simulink model "l1ipswing"  (Simulink 5.0)
settings: Solver=ode1  SolverMode=SingleTasking  StartTime=0.0  StopTime=inf  FixedStep=0.005  RelTol=1e-3
settings Model: LastModifiedBy=Administrator  ExtModeMexFile=rtwinext  ExtModeTrigDuration=100000  SimulationMode=external  LimitDataPoints=off  MaxDataPoints=20000  RTWSystemTargetFile=rtwin.tlc  RTWTemplateMakefile=rtwintmf  RTWOptions="-aCCOptimize=1 -aEnforceIntegerDowncast=1 -aExtMode=1 -aFoldNonRolledExpr=1 -aForceParamTrailComments=0 -aGenerateComments=1 -aGenerateReport=0 -aIncDataTypeInIds=0 -aIncHierarchyInIds=0 -aInlineInvariantSignals=0 -aInlineParameters=0 -aInlinedPrmAccess=\"Literals\" -aLocalBlockOutputs=1 -aMaxRTWIdLen=31 -aPrefixModelToSubsysFcnNames=1 -aRTWVerbose=1 -aRebuildAll=0 -aRollThreshold=5 -aShowEliminatedStatements=0"

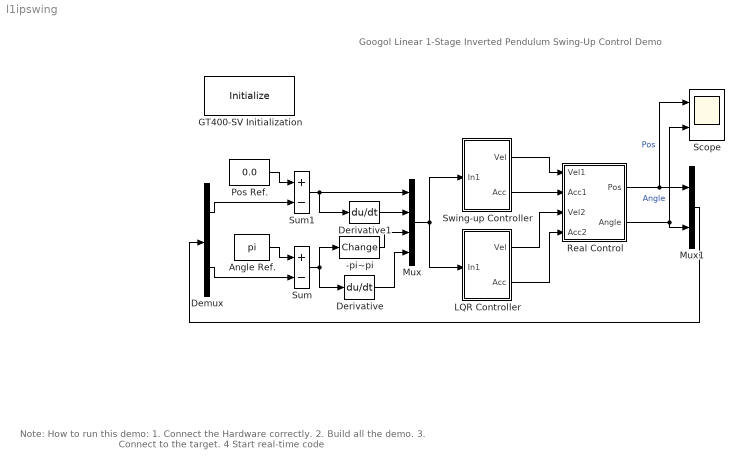
== system l1ipswing ==
  note: Googol Linear 1-Stage Inverted Pendulum Swing-Up Control Demo
  note: Note:
      |          How to run this demo:
      |          1.  Connect the Hardware correctly.
      |          2.  Build all the demo.
      |          3.  Connect to the target.
      |          4  Start real-time code
  " -pi~pi" : S-Function  AncestorBlock=googolbox/GT-400-SV Block Library/ -pi~pi  FunctionName=Change
      mask Type: Change
      mask Description:
      | Change input signal between -pi and pi in 2*pi period.
      | Block input:
      |     any double.
      | Block output:
      |     between -pi and pi.
      | eg:
      |     If input is 1.5*pi, then output is -0.5*pi.
      mask Help:
      | This block, "change", input signal between -pi and pi in 2*pi period.
      | Block input:
      |     any double.
      | Block output:
      |     between -pi and pi.
      | eg:
      |     input is 1.5*pi, then output is -0.5*pi.
      mask Display: plot([0:0.01:2*pi],sin([0:0.01:2*pi]));
  Angle Ref. : Constant  Value=pi
  Demux : Demux  Outputs=2
  Derivative : Derivative
  Derivative1 : Derivative
  GT400-SV Initialization : S-Function  Priority=0  AncestorBlock=googolbox/GT-400-SV Block Library/GT400-SV Initialization  FunctionName=Initialize  Parameters=openloop  mask(Initialize){openloop=0}
      mask prompts: openloop "Control loop:"
      mask help:
      | Initializing the googol GT400-SV motion control board.
      | Block parameter:
      |     Control loop:
      |          0: closed-loop control.
      |          1: opened-loop control.
      mask Help: This initialize block initializes the googol GT400-SV motion control board.
      mask Display: disp('Initialize \nGT400-SV');
  LQR Controller : Subsystem  mask{x=-31.62, xdot=-20.95, angle=77.8, angledot=11.76}
      mask prompts: x "Kx"; xdot "Kx'"; angle "Ka"; angledot "Ka'"
  Mux : Mux
  Mux1 : Mux  Inputs=2
  Pos Ref. : Constant  Value=0.0
  Real Control : Subsystem
  Scope : Scope  NumInputPorts=2
      settings: TickLabels=on  TimeRange=50  YMin=-0.3~-3  YMax=0.1~4  MaxDataPoints=20000
  Sum : Sum  Inputs=+-  SaturateOnIntegerOverflow=on
  Sum1 : Sum  Inputs=+-  SaturateOnIntegerOverflow=on
  Swing-up Controller : Subsystem
  wires:
  Mux/1 -> LQR Controller/1(In1), Swing-up Controller/1(In1)
  Real Control/1(Pos) -> Mux1/1, Scope/1  "Pos"
  Mux1/1 -> Demux/1
  Sum/1 -> Derivative/1, " -pi~pi"/1
  Derivative/1 -> Mux/4
  LQR Controller/2(Acc) -> Real Control/4(Acc2)
  Swing-up Controller/2(Acc) -> Real Control/2(Acc1)
  Demux/1 -> Sum1/2
  Sum1/1 -> Derivative1/1, Mux/1
  Pos Ref./1 -> Sum1/1
  Swing-up Controller/1(Vel) -> Real Control/1(Vel1)
  Angle Ref./1 -> Sum/1
  Demux/2 -> Sum/2
  " -pi~pi"/1 -> Mux/3
  Derivative1/1 -> Mux/2
  Real Control/2(Angle) -> Mux1/2, Scope/2  "Angle"
  LQR Controller/1(Vel) -> Real Control/3(Vel2)

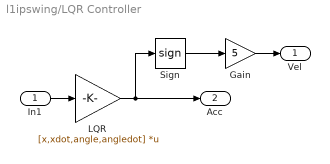
== system l1ipswing/LQR Controller ==
  In1 : Inport
  Gain : Gain  Gain=5  SaturateOnIntegerOverflow=on
  LQR : Gain  Gain=[x,xdot,angle,angledot]  Multiplication=Matrix(K*u)  SaturateOnIntegerOverflow=on
  Sign : Signum
  Vel : Outport
  Acc : Outport  Port=2
  wires:
  LQR/1 -> Sign/1, Acc/1
  Sign/1 -> Gain/1
  Gain/1 -> Vel/1
  In1/1 -> LQR/1

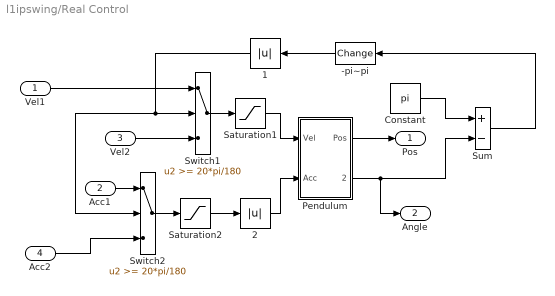
== system l1ipswing/Real Control ==
  Vel1 : Inport
  Acc1 : Inport  Port=2
  Vel2 : Inport  Port=3
  Acc2 : Inport  Port=4
  " -pi~pi" : S-Function  Orientation=left  AncestorBlock=googolbox/GT-400-SV Block Library/ -pi~pi  FunctionName=Change
      mask Type: Change
      mask Description:
      | Change input signal between -pi and pi in 2*pi period.
      | Block input:
      |     any double.
      | Block output:
      |     between -pi and pi.
      | eg:
      |     If input is 1.5*pi, then output is -0.5*pi.
      mask Help:
      | This block, "change", input signal between -pi and pi in 2*pi period.
      | Block input:
      |     any double.
      | Block output:
      |     between -pi and pi.
      | eg:
      |     input is 1.5*pi, then output is -0.5*pi.
      mask Display: plot([0:0.01:2*pi],sin([0:0.01:2*pi]));
  " 1" : Abs  Orientation=left  SaturateOnIntegerOverflow=on
  " 2" : Abs  SaturateOnIntegerOverflow=on
  Constant : Constant  Value=pi
  Pendulum : Subsystem
  Saturation1 : Saturate  UpperLimit=1.5  LowerLimit=-1.5
  Saturation2 : Saturate  UpperLimit=15  LowerLimit=-15
  Sum : Sum  Inputs=+-  SaturateOnIntegerOverflow=on
  Switch1 : Switch  Threshold=20*pi/180  SaturateOnIntegerOverflow=on
  Switch2 : Switch  Threshold=20*pi/180  SaturateOnIntegerOverflow=on
  Pos : Outport
  Angle : Outport  Port=2
  wires:
  Switch2/1 -> Saturation2/1
  " 2"/1 -> Pendulum/2(Acc)
  " 1"/1 -> Switch1/2, Switch2/2
  Vel1/1 -> Switch1/1
  Pendulum/1(Pos) -> Pos/1
  Acc1/1 -> Switch2/1
  Constant/1 -> Sum/1
  Sum/1 -> " -pi~pi"/1
  Saturation2/1 -> " 2"/1
  Acc2/1 -> Switch2/3
  Vel2/1 -> Switch1/3
  Switch1/1 -> Saturation1/1
  Pendulum/2(Angle) -> Sum/2, Angle/1
  " -pi~pi"/1 -> " 1"/1
  Saturation1/1 -> Pendulum/1(Vel)

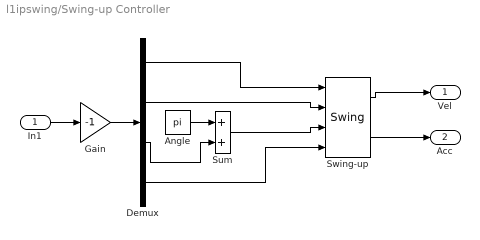
== system l1ipswing/Swing-up Controller ==
  In1 : Inport
  Angle : Constant  Value=pi
  Demux : Demux
  Gain : Gain  Gain=-1  SaturateOnIntegerOverflow=on
  Sum : Sum  SaturateOnIntegerOverflow=on
  Swing-up : S-Function  FunctionName=Swing  Parameters=energycof  mask{energycof=0.159}
      mask prompts: energycof "Energy Coefficient"
  Vel : Outport
  Acc : Outport  Port=2
  wires:
  In1/1 -> Gain/1
  Swing-up/1 -> Vel/1
  Angle/1 -> Sum/1
  Swing-up/2 -> Acc/1
  Demux/3 -> Sum/2
  Sum/1 -> Swing-up/3
  Demux/4 -> Swing-up/4
  Demux/2 -> Swing-up/2
  Demux/1 -> Swing-up/1
  Gain/1 -> Demux/1

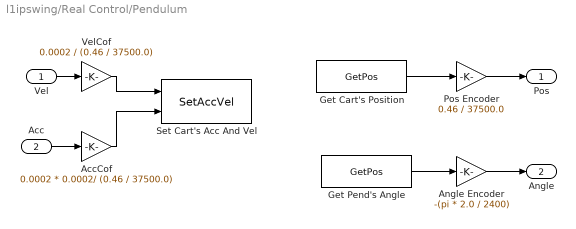
== system l1ipswing/Real Control/Pendulum ==
  Vel : Inport
  Acc : Inport  Port=2
  AccCof : Gain  Gain=0.0002 * 0.0002/ (0.46 / 37500.0)  SaturateOnIntegerOverflow=on
  Angle Encoder : Gain  Gain=-(pi * 2.0 / 2400)  SaturateOnIntegerOverflow=on
  Get Cart's Position : S-Function  Priority=1  AncestorBlock=googolbox/GT-400-SV Block Library/Get Current Axis' Position  FunctionName=GetPos  Parameters=axis  mask(GetPos){axis=1}
      mask prompts: axis "Axis number:"
      mask help:
      | Getting the current axis position value in encoder' counts.
      | Block parameter:
      |     Axis number:  must be between 1 and 6, default is 1.
      | Block output:
      |     1~4: current axis' encoder reading counts.
      |     5/6: assistant encoder 1/2 reading counts.
      mask Help:
      | This block, GetPos, is intended for getting the current axis position value in encoder' counts. This value represents the actual position for the axis
      | at the current sample time. This command operates for all profile modes.
      | The value returned is a 32-bit signed number with units of counts.
      | The range is -1,073,741,824 to 1,073,741,823.
      | 
      | You can recalculate obtained value into meter units via multiplication by the scaler coefficient .
      | 
      | Block parameter:
      |     Axis number:  must be between 1 and 4, default is 1.
      | Block input: none.
      | Block output:
      |         1~4: current axis' encoder reading counts.
      |         5/6: assistant encoder 1/2 reading counts.
      mask Display:
      | disp('GetPos');
      | port_label('output', 1, 'Pos');
  Get Pend's Angle : S-Function  Priority=1  AncestorBlock=googolbox/GT-400-SV Block Library/Get Current Axis' Position  FunctionName=GetPos  Parameters=axis  mask(GetPos){axis=2}
      mask prompts: axis "Axis number:"
      mask help:
      | Getting the current axis position value in encoder' counts.
      | Block parameter:
      |     Axis number:  must be between 1 and 6, default is 1.
      | Block output:
      |     1~4: current axis' encoder reading counts.
      |     5/6: assistant encoder 1/2 reading counts.
      mask Help:
      | This block, GetPos, is intended for getting the current axis position value in encoder' counts. This value represents the actual position for the axis
      | at the current sample time. This command operates for all profile modes.
      | The value returned is a 32-bit signed number with units of counts.
      | The range is -1,073,741,824 to 1,073,741,823.
      | 
      | You can recalculate obtained value into meter units via multiplication by the scaler coefficient .
      | 
      | Block parameter:
      |     Axis number:  must be between 1 and 4, default is 1.
      | Block input: none.
      | Block output:
      |         1~4: current axis' encoder reading counts.
      |         5/6: assistant encoder 1/2 reading counts.
      mask Display:
      | disp('GetPos');
      | port_label('output', 1, 'Pos');
  Pos Encoder : Gain  Gain=0.46 / 37500.0  SaturateOnIntegerOverflow=on
  Set Cart's Acc And Vel : S-Function  Priority=1  AncestorBlock=googolbox/GT-400-SV Block Library/Set Current Axis' Acc and Vel  FunctionName=SetAccVel  Parameters=axis, vel, pos  mask(SetAccVel){axis=1, vel=0.1, pos=250000}
      mask prompts: axis "Axis number:"; vel "Back velocity:"; pos "Back position:"
      mask help:
      | Setting the current axis' acceleration and velocity.
      |
      | Block parameter:
      |     Axis number:
      |         must be between 1 and 4, default is 1;
      |     Back velocity:
      |          After the current axis' limit reached, the moter will moves back as this  velocity, it must >=0;
      |     Back position:
      |          After the current axis' limit reached, the moter will moves back to this postion relative to limit, it must >=0;
      |
      | Block input:
      |     Vel: the current axis' velocity.
      |     Acc: the current axis' acceleration.
      mask Help:
      | This SetAccVel bolck Sets the current axis' acceleration and velocity.
      | Block parameter:
      |     Axis number: must be between 1 and 4, default is 1.
      | Block input:
      |     Vel: the current axis' velocity.
      |     Acc: the current axis' acceleration.
      mask Display:
      | disp('          SetAccVel');
      | port_label('input', 1, 'Vel');
      | port_label('input', 2, 'Acc');
  VelCof : Gain  Gain=0.0002 / (0.46 / 37500.0)  SaturateOnIntegerOverflow=on
  Pos : Outport
  Angle : Outport  Port=2
  wires:
  Angle Encoder/1 -> Angle/1
  Pos Encoder/1 -> Pos/1
  Get Pend's Angle/1 -> Angle Encoder/1
  Acc/1 -> AccCof/1
  Vel/1 -> VelCof/1
  Get Cart's Position/1 -> Pos Encoder/1
  AccCof/1 -> Set Cart's Acc And Vel/2
  VelCof/1 -> Set Cart's Acc And Vel/1
